simulink model "framework_sim_r2018b"  (R2018b)
settings: Solver=FixedStepAuto  SolverName=FixedStepDiscrete  StartTime=T0  StopTime=Tf  FixedStep=Ts  EnableMultiTasking=on
model workspace (MAT data in the model file):
  aKalman = Simulink.Parameter
  aKalman.DataType = 'auto'
  aKalman.Dimensions = [0 0]
  slipEnabler = Simulink.Parameter
  slipEnabler.DataType = 'auto'
  slipEnabler.Dimensions = [0 0]
values from neighbouring files (symbols this model uses):
  enable_onlinePlots = 0    [main_framework.m]
  enable_zoom = 1    [main_framework.m]
  LLC_sampleTime = LLC.sample_time    [main_framework.m]
  longCTRparam = longitController()    [main_framework.m]
  mapObjects = scenario.scenario_data.mapObjects    [main_framework.m]
  pacejkaParam = loadPacejkaParam()    [main_framework.m]
  refRoute_fewPoints = referencePath_fewPoints.refRoute_fewPoints    [main_framework.m]
  tau_D = vehicle_data.steering_system.tau_D    [main_framework.m]
  Ts = simulationPars.times.step_size    [main_framework.m]
  vehicle_data = getVehicleDataStruct()    [main_framework.m]
  X0 = loadInitialConditions    [main_framework.m]
undefined symbols (not defined in the file or in its folder): DiscIntNeverNeededParam, latContr_select
libraries: simulink_extras x13, drivingvehiclecontroller x2, simulink x1
settings Model: Creator=Edoardo  LastModifiedBy=tonegas
settings DataIOCC: SaveFormat=Array  ReturnWorkspaceOutputs=on
settings OptimizationCC: DefaultParameterBehavior=Inlined  PassReuseOutputArgsAs=Individual arguments  MaxStackSize=64
settings DebuggingCC: ReadBeforeWriteMsg=DisableAll  WriteAfterWriteMsg=DisableAll  WriteAfterReadMsg=DisableAll  MultiTaskDSMMsg=none  ParameterTunabilityLossMsg=error  SFUnexpectedBacktrackingDiag=warning  SFNoUnconditionalDefaultTransitionDiag=warning  SFExecutionAtInitializationDiag=none
settings HardwareCC: ProdBitPerInt=16  ProdBitPerPointer=16  ProdBitPerSizeT=16  ProdBitPerPtrDiffT=16  ProdLargestAtomicFloat=None  ProdWordSize=16  ProdHWDeviceType=STMicroelectronics->ST10/Super10
settings ModelReferenceCC: UpdateModelReferenceTargets=IfOutOfDate  PropagateSignalLabelsOutOfModel=off
settings SFSimCC: SFSimEcho=off  SimUseLocalCustomCode=off  MATLABDynamicMemAlloc=off
settings RTWCC: SystemTargetFile=ert.tlc  TemplateMakefile=ert_default_tmf  GenerateReport=on  RetainRTWFile=on  RTWUseLocalCustomCode=off  Toolchain=GNU Tools for ARM Embedded Processors  BuildConfiguration=Faster Runs  IncludeHyperlinkInReport=on  LaunchReport=on  GenerateTraceInfo=on  GenerateTraceReport=on  GenerateTraceReportSl=on  GenerateTraceReportSf=on  GenerateTraceReportEml=on
settings CodeAppCC: ForceParamTrailComments=on  IgnoreCustomStorageClasses=off  OperatorAnnotations=on  SimulinkDataObjDesc=on  SFDataObjDesc=on  InsertBlockDesc=on
settings ERTTargetCC: CodeReplacementLibrary=ARM Cortex-M (Optimized)  SupportVariableSizeSignals=on  RootIOFormat=Structure reference  ERTCustomFileTemplate=example_file_process.tlc
settings ConfigComp: CovMetricSettings=dw  CovSaveCumulativeToWorkspaceVar=on  CovSaveSingleToWorkspaceVar=on  CovExternalEMLEnable=off

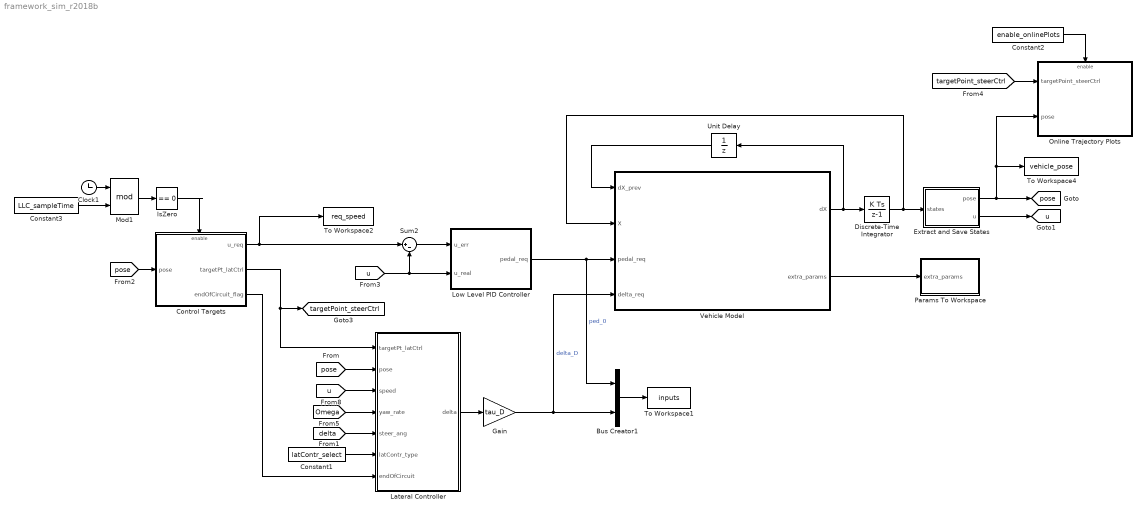
== system framework_sim_r2018b ==
  Bus Creator1 : BusCreator  Inputs=2
  Clock1 : Clock
  Constant1 : Constant  Value=latContr_select
  Constant2 : Constant  Value=enable_onlinePlots
  Constant3 : Constant  Value=LLC_sampleTime
  Control Targets : Subsystem
  Discrete-Time Integrator : DiscreteIntegrator  gainval=1  InitialCondition=X0  SampleTime=-1  ICPrevOutput=DiscIntNeverNeededParam  ICPrevScaledInput=DiscIntNeverNeededParam
  Extract and Save States : Subsystem
  Gain : Gain  Gain=tau_D
  IsZero : simulink/Logic and Bit Operations/Compare To Zero  relop===  OutDataTypeStr=boolean
  Lateral Controller : Subsystem
  Low Level PID Controller : Subsystem
  Mod1 : Math  Operator=mod  SaturateOnIntegerOverflow=on
  Online Trajectory Plots : Subsystem
      mask Display: image('example_path.png'); % Use "Edit Image" on toolstrip to change.
  Params To Workspace : Subsystem
  Sum2 : Sum  Inputs=|+-
  To Workspace1 : ToWorkspace  VariableName=inputs  SaveFormat=Timeseries  SampleTime=-1
  To Workspace2 : ToWorkspace  VariableName=req_speed  SaveFormat=Timeseries  SampleTime=-1
  To Workspace4 : ToWorkspace  VariableName=vehicle_pose  SampleTime=-1
      settings: Save2DSignal=2-D array (concatenate along first dimension)
  Unit Delay : UnitDelay  InitialCondition=zeros(size(X0))  SampleTime=-1  HasFrameUpgradeWarning=on
  Vehicle Model : MATLAB Function  TreatAsAtomicUnit=on
  tag scope: pose=global, targetPoint_steerCtrl=global, u=global
  wires:
  [targetPoint_steerCtrl] -> Online Trajectory Plots/1(targetPoint_steerCtrl)
  Constant2/1 -> Online Trajectory Plots/Enable
  [pose] -> Lateral Controller/2(pose)
  [u] -> Lateral Controller/3(speed)
  Constant1/1 -> Lateral Controller/6(latContr_type)
  [Omega] -> Lateral Controller/4(yaw_rate)
  [delta] -> Lateral Controller/5(steer_ang)
  Control Targets/2(targetPt_latCtrl) -> Lateral Controller/1(targetPt_latCtrl), [targetPoint_steerCtrl]
  [pose] -> Control Targets/1(pose)
  Clock1/1 -> Mod1/1
  Constant3/1 -> Mod1/2
  Mod1/1 -> IsZero/1
  IsZero/1 -> Control Targets/Enable
  Control Targets/3(endOfCircuit_flag) -> Lateral Controller/7(endOfCircuit)
  Unit Delay/1 -> Vehicle Model/1(dX_prev)
  Discrete-Time Integrator/1 -> Extract and Save States/1(states), Vehicle Model/2(X)
  Sum2/1 -> Low Level PID Controller/1(u_err)
  Gain/1 -> Bus Creator1/2, Vehicle Model/4(delta_req)  "delta_D"
  Control Targets/1(u_req) -> Sum2/1, To Workspace2/1
  Vehicle Model/1(dX) -> Unit Delay/1, Discrete-Time Integrator/1
  Vehicle Model/2(extra_params) -> Params To Workspace/1(extra_params)
  Bus Creator1/1 -> To Workspace1/1
  Low Level PID Controller/1(pedal_req) -> Vehicle Model/3(pedal_req), Bus Creator1/1  "ped_0"
  Lateral Controller/1(delta) -> Gain/1
  Extract and Save States/1(pose) -> [pose], Online Trajectory Plots/2(pose), To Workspace4/1
  Extract and Save States/2(u) -> [u]
  [u] -> Sum2/2, Low Level PID Controller/2(u_real)

== system framework_sim_r2018b/Control Targets ==
  pose : Inport
  Enable : EnablePort
  MATLAB System : MATLABSystem  System=setControlTargets  lateralController_type=latContr_select  purePursuit_lookAhead=purePursuitParams.lookAhead  clothoidBased_lookAhead=clothoidBasedParams.lookAhead  refRoute_points=refRoute_fewPoints  Lf=vehicle_data.vehicle.Lf  x_parkLot=mapObjects(1,1)  y_lowBound_parkLot=mapObjects(2,2)  y_uppBound_parkLot=mapObjects(1,2)  SimulateUsing=Interpreted execution
      mask Type: setControlTargets
      mask Display:
      | disp('setControlTargets');
      | port_label('input',1,'vehPose');
      | port_label('output',1,'targetPoint_latControl');
      | port_label('output',2,'speed_req');
      | port_label('output',3,'endOfCircuit');
  u_req : Outport  VectorParamsAs1DForOutWhenUnconnected=off
  targetPt_latCtrl : Outport  Port=2  VectorParamsAs1DForOutWhenUnconnected=off
  endOfCircuit_flag : Outport  Port=3  VectorParamsAs1DForOutWhenUnconnected=off
  wires:
  pose/1 -> MATLAB System/1
  MATLAB System/2 -> u_req/1
  MATLAB System/1 -> targetPt_latCtrl/1
  MATLAB System/3 -> endOfCircuit_flag/1

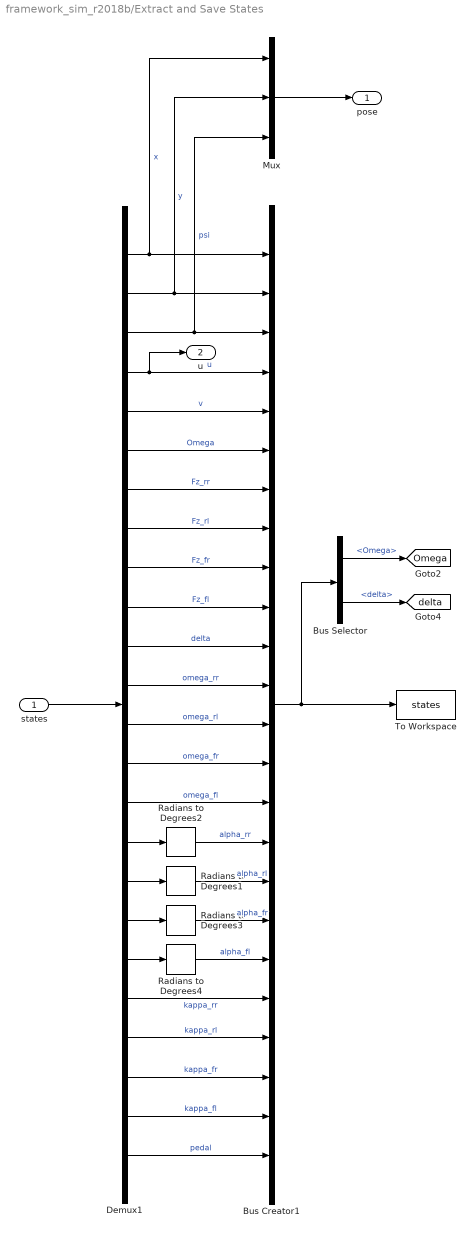
== system framework_sim_r2018b/Extract and Save States ==
  states : Inport
  Bus Creator1 : BusCreator  Inputs=24
  Bus Selector : BusSelector  OutputSignals=Omega,delta
  Demux1 : Demux  Outputs=24
  Mux : Mux  Inputs=3
  Radians to Degrees{1..4} (4 alike) : simulink_extras/Transformations/Radians to Degrees
  To Workspace : ToWorkspace  VariableName=states  SaveFormat=Timeseries  SampleTime=-1
  pose : Outport
  u : Outport  Port=2
  tag scope: Omega=global, delta=global
  wires:
  Demux1/13 -> Bus Creator1/13  "omega_rl"
  Demux1/8 -> Bus Creator1/8  "Fz_rl"
  Demux1/23 -> Bus Creator1/23  "kappa_fl"
  Demux1/19 -> Radians to Degrees4/1
  states/1 -> Demux1/1
  Demux1/14 -> Bus Creator1/14  "omega_fr"
  Demux1/7 -> Bus Creator1/7  "Fz_rr"
  Demux1/15 -> Bus Creator1/15  "omega_fl"
  Demux1/3 -> Mux/3, Bus Creator1/3  "psi"
  Demux1/22 -> Bus Creator1/22  "kappa_fr"
  Demux1/4 -> Bus Creator1/4, u/1  "u"
  Demux1/6 -> Bus Creator1/6  "Omega"
  Demux1/11 -> Bus Creator1/11  "delta"
  Demux1/5 -> Bus Creator1/5  "v"
  Demux1/9 -> Bus Creator1/9  "Fz_fr"
  Demux1/21 -> Bus Creator1/21  "kappa_rl"
  Demux1/12 -> Bus Creator1/12  "omega_rr"
  Demux1/17 -> Radians to Degrees1/1
  Demux1/2 -> Mux/2, Bus Creator1/2  "y"
  Demux1/20 -> Bus Creator1/20  "kappa_rr"
  Demux1/10 -> Bus Creator1/10  "Fz_fl"
  Demux1/18 -> Radians to Degrees3/1
  Demux1/1 -> Mux/1, Bus Creator1/1  "x"
  Demux1/16 -> Radians to Degrees2/1
  Bus Creator1/1 -> Bus Selector/1, To Workspace/1
  Radians to Degrees2/1 -> Bus Creator1/16  "alpha_rr"
  Radians to Degrees1/1 -> Bus Creator1/17  "alpha_rl"
  Radians to Degrees3/1 -> Bus Creator1/18  "alpha_fr"
  Radians to Degrees4/1 -> Bus Creator1/19  "alpha_fl"
  Demux1/24 -> Bus Creator1/24  "pedal"
  Mux/1 -> pose/1
  Bus Selector/1 -> [Omega]  "<Omega>"
  Bus Selector/2 -> [delta]  "<delta>"

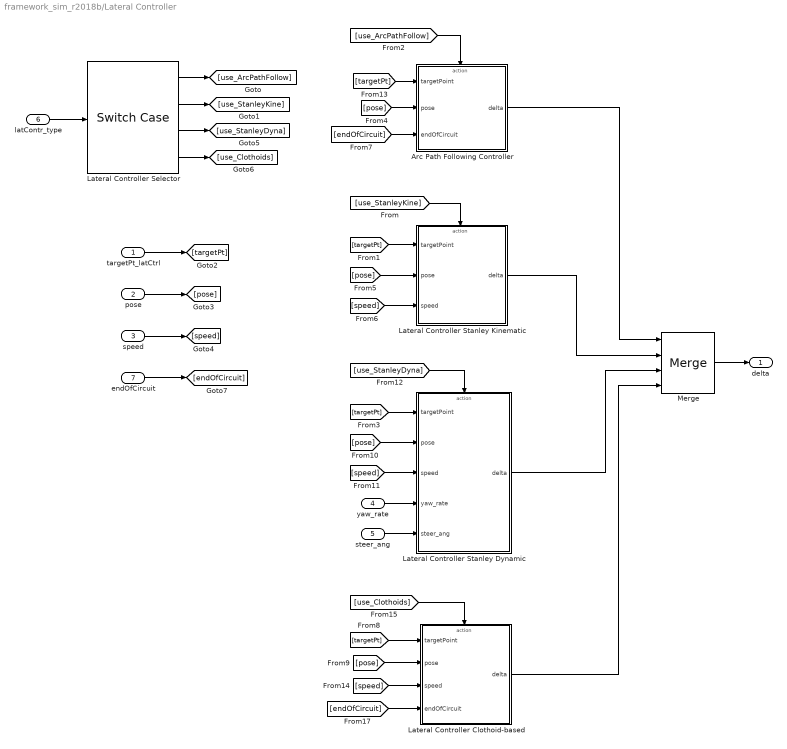
== system framework_sim_r2018b/Lateral Controller ==
  targetPt_latCtrl : Inport
  pose : Inport  Port=2
  speed : Inport  Port=3
  yaw_rate : Inport  Port=4
  steer_ang : Inport  Port=5
  latContr_type : Inport  Port=6
  endOfCircuit : Inport  Port=7
  Arc Path Following Controller : Subsystem  TreatAsAtomicUnit=on
  Lateral Controller Clothoid-based : Subsystem  TreatAsAtomicUnit=on
  Lateral Controller Selector : SwitchCase  CaseConditions={1,2,3,4}  ShowDefaultCase=off
  Lateral Controller Stanley Dynamic : Subsystem  TreatAsAtomicUnit=on
  Lateral Controller Stanley Kinematic : Subsystem  TreatAsAtomicUnit=on
  Merge : Merge  Inputs=4
  delta : Outport  VectorParamsAs1DForOutWhenUnconnected=off
  wires:
  Arc Path Following Controller/1(delta) -> Merge/1
  latContr_type/1 -> Lateral Controller Selector/1
  Lateral Controller Stanley Kinematic/1(delta) -> Merge/2
  Merge/1 -> delta/1
  Lateral Controller Selector/1 -> [use_ArcPathFollow]
  [use_ArcPathFollow] -> Arc Path Following Controller/Action
  Lateral Controller Selector/2 -> [use_StanleyKine]
  [use_StanleyKine] -> Lateral Controller Stanley Kinematic/Action
  targetPt_latCtrl/1 -> [targetPt]
  [targetPt] -> Arc Path Following Controller/1(targetPoint)
  [targetPt] -> Lateral Controller Stanley Kinematic/1(targetPoint)
  pose/1 -> [pose]
  [pose] -> Arc Path Following Controller/2(pose)
  [pose] -> Lateral Controller Stanley Kinematic/2(pose)
  speed/1 -> [speed]
  [speed] -> Lateral Controller Stanley Kinematic/3(speed)
  Lateral Controller Selector/3 -> [use_StanleyDyna]
  [pose] -> Lateral Controller Stanley Dynamic/2(pose)
  [targetPt] -> Lateral Controller Stanley Dynamic/1(targetPoint)
  [speed] -> Lateral Controller Stanley Dynamic/3(speed)
  [use_StanleyDyna] -> Lateral Controller Stanley Dynamic/Action
  Lateral Controller Stanley Dynamic/1(delta) -> Merge/3
  yaw_rate/1 -> Lateral Controller Stanley Dynamic/4(yaw_rate)
  steer_ang/1 -> Lateral Controller Stanley Dynamic/5(steer_ang)
  [use_Clothoids] -> Lateral Controller Clothoid-based/Action
  [pose] -> Lateral Controller Clothoid-based/2(pose)
  [targetPt] -> Lateral Controller Clothoid-based/1(targetPoint)
  [speed] -> Lateral Controller Clothoid-based/3(speed)
  Lateral Controller Clothoid-based/1(delta) -> Merge/4
  Lateral Controller Selector/4 -> [use_Clothoids]
  [endOfCircuit] -> Arc Path Following Controller/3(endOfCircuit)
  [endOfCircuit] -> Lateral Controller Clothoid-based/4(endOfCircuit)
  endOfCircuit/1 -> [endOfCircuit]

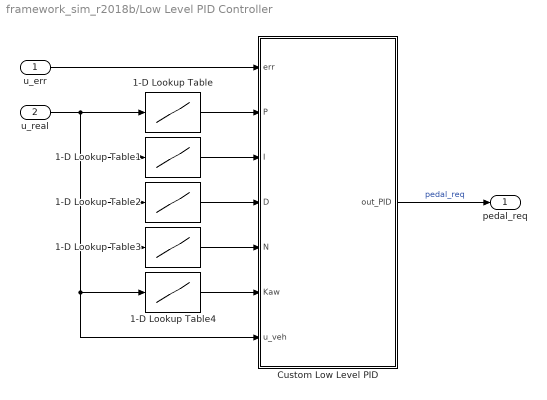
== system framework_sim_r2018b/Low Level PID Controller ==
  u_err : Inport
  u_real : Inport  Port=2
  1-D Lookup Table : Lookup_n-D  NumberOfTableDimensions=1  BreakpointsForDimension1=longCTRparam.speed_vals_PID_sched  BeginIndexSearchUsingPreviousIndexResult=on  Table=longCTRparam.Kp_vals  ExtrapMethod=Clip  UseLastTableValue=on  InternalRulePriority=Speed  RndMeth=Simplest  InputSameDT=on
  1-D Lookup Table1 : Lookup_n-D  NumberOfTableDimensions=1  BreakpointsForDimension1=longCTRparam.speed_vals_PID_sched  BeginIndexSearchUsingPreviousIndexResult=on  Table=longCTRparam.Ki_vals  ExtrapMethod=Clip  UseLastTableValue=on  InternalRulePriority=Speed  RndMeth=Simplest  InputSameDT=on
  1-D Lookup Table2 : Lookup_n-D  NumberOfTableDimensions=1  BreakpointsForDimension1=longCTRparam.speed_vals_PID_sched  BeginIndexSearchUsingPreviousIndexResult=on  Table=longCTRparam.Kd_vals  ExtrapMethod=Clip  UseLastTableValue=on  InternalRulePriority=Speed  RndMeth=Simplest  InputSameDT=on
  1-D Lookup Table3 : Lookup_n-D  NumberOfTableDimensions=1  BreakpointsForDimension1=longCTRparam.speed_vals_PID_sched  BeginIndexSearchUsingPreviousIndexResult=on  Table=longCTRparam.N_vals  ExtrapMethod=Clip  UseLastTableValue=on  InternalRulePriority=Speed  RndMeth=Simplest  InputSameDT=on
  1-D Lookup Table4 : Lookup_n-D  NumberOfTableDimensions=1  BreakpointsForDimension1=longCTRparam.speed_vals_PID_sched  BeginIndexSearchUsingPreviousIndexResult=on  Table=longCTRparam.Kaw_vals  ExtrapMethod=Clip  UseLastTableValue=on  InternalRulePriority=Speed  RndMeth=Simplest  InputSameDT=on
  Custom Low Level PID : Subsystem
  pedal_req : Outport  VectorParamsAs1DForOutWhenUnconnected=off
  wires:
  1-D Lookup Table/1 -> Custom Low Level PID/2(P)
  u_err/1 -> Custom Low Level PID/1(err)
  u_real/1 -> 1-D Lookup Table4/1, Custom Low Level PID/7(u_veh), 1-D Lookup Table3/1, 1-D Lookup Table2/1, 1-D Lookup Table1/1, 1-D Lookup Table/1
  1-D Lookup Table2/1 -> Custom Low Level PID/4(D)
  1-D Lookup Table3/1 -> Custom Low Level PID/5(N)
  1-D Lookup Table1/1 -> Custom Low Level PID/3(I)
  Custom Low Level PID/1(out_PID) -> pedal_req/1  "pedal_req"
  1-D Lookup Table4/1 -> Custom Low Level PID/6(Kaw)

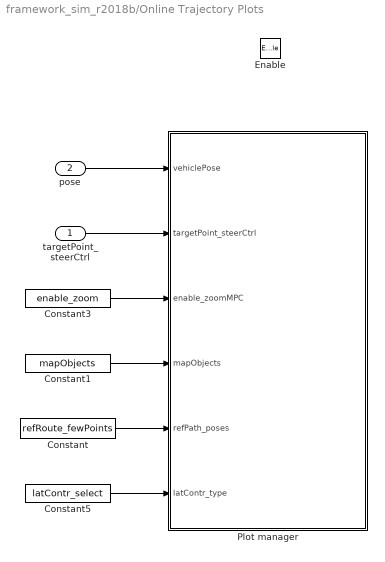
== system framework_sim_r2018b/Online Trajectory Plots ==
  targetPoint_steerCtrl : Inport
  pose : Inport  Port=2
  Enable : EnablePort
  Constant : Constant  Value=refRoute_fewPoints
  Constant1 : Constant  Value=mapObjects
  Constant3 : Constant  Value=enable_zoom
  Constant5 : Constant  Value=latContr_select
  Plot manager : MATLAB Function  TreatAsAtomicUnit=on
  wires:
  Constant1/1 -> Plot manager/4(mapObjects)
  targetPoint_steerCtrl/1 -> Plot manager/2(targetPoint_steerCtrl)
  Constant5/1 -> Plot manager/6(latContr_type)
  Constant/1 -> Plot manager/5(refPath_poses)
  pose/1 -> Plot manager/1(vehiclePose)
  Constant3/1 -> Plot manager/3(enable_zoomMPC)

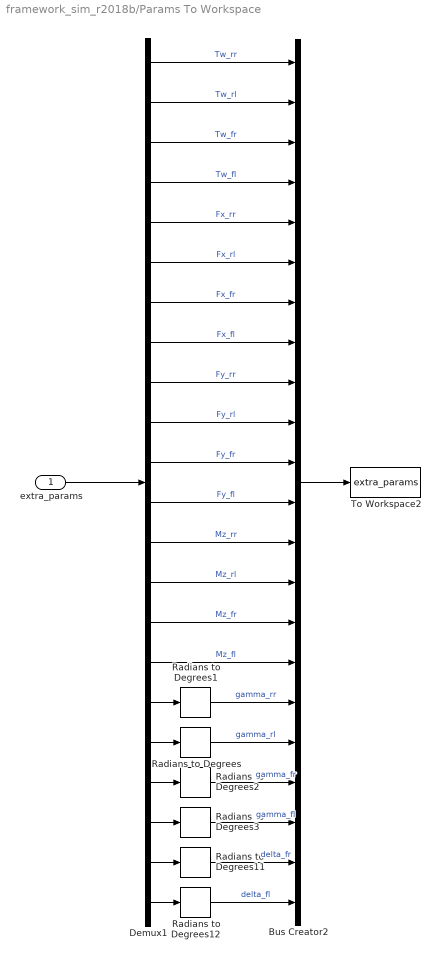
== system framework_sim_r2018b/Params To Workspace ==
  extra_params : Inport
  Bus Creator2 : BusCreator  Inputs=22
  Demux1 : Demux  Outputs=22
  Radians to Degrees{,1..3,11..12} (6 alike) : simulink_extras/Transformations/Radians to Degrees
  To Workspace2 : ToWorkspace  VariableName=extra_params  SaveFormat=Timeseries  SampleTime=-1
  wires:
  Demux1/17 -> Radians to Degrees1/1
  Demux1/3 -> Bus Creator2/3  "Tw_fr"
  Radians to Degrees3/1 -> Bus Creator2/20  "gamma_fl"
  Demux1/16 -> Bus Creator2/16  "Mz_fl"
  Radians to Degrees1/1 -> Bus Creator2/17  "gamma_rr"
  Radians to Degrees11/1 -> Bus Creator2/21  "delta_fr"
  Demux1/14 -> Bus Creator2/14  "Mz_rl"
  Demux1/4 -> Bus Creator2/4  "Tw_fl"
  Demux1/6 -> Bus Creator2/6  "Fx_rl"
  Demux1/8 -> Bus Creator2/8  "Fx_fl"
  Demux1/13 -> Bus Creator2/13  "Mz_rr"
  Demux1/7 -> Bus Creator2/7  "Fx_fr"
  Demux1/5 -> Bus Creator2/5  "Fx_rr"
  Demux1/9 -> Bus Creator2/9  "Fy_rr"
  Demux1/11 -> Bus Creator2/11  "Fy_fr"
  Demux1/15 -> Bus Creator2/15  "Mz_fr"
  Demux1/10 -> Bus Creator2/10  "Fy_rl"
  Radians to Degrees12/1 -> Bus Creator2/22  "delta_fl"
  Radians to Degrees2/1 -> Bus Creator2/19  "gamma_fr"
  extra_params/1 -> Demux1/1
  Demux1/12 -> Bus Creator2/12  "Fy_fl"
  Bus Creator2/1 -> To Workspace2/1
  Demux1/1 -> Bus Creator2/1  "Tw_rr"
  Demux1/2 -> Bus Creator2/2  "Tw_rl"
  Radians to Degrees/1 -> Bus Creator2/18  "gamma_rl"
  Demux1/18 -> Radians to Degrees/1
  Demux1/19 -> Radians to Degrees2/1
  Demux1/20 -> Radians to Degrees3/1
  Demux1/21 -> Radians to Degrees11/1
  Demux1/22 -> Radians to Degrees12/1

== system framework_sim_r2018b/Lateral Controller/Arc Path Following Controller ==
  targetPoint : Inport
  pose : Inport  Port=2
  endOfCircuit : Inport  Port=3
  Action Port : ActionPort
  Arc Path Following Controller : MATLAB Function  TreatAsAtomicUnit=on
  delta : Outport  VectorParamsAs1DForOutWhenUnconnected=off
  wires:
  Arc Path Following Controller/1(delta) -> delta/1
  targetPoint/1 -> Arc Path Following Controller/1(target_Point)
  pose/1 -> Arc Path Following Controller/2(pose)
  endOfCircuit/1 -> Arc Path Following Controller/3(endOfCircuit)

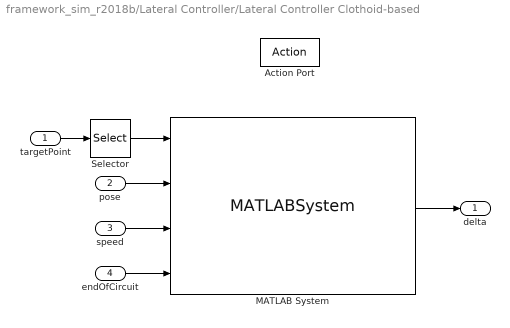
== system framework_sim_r2018b/Lateral Controller/Lateral Controller Clothoid-based ==
  targetPoint : Inport
  pose : Inport  Port=2
  speed : Inport  Port=3
  endOfCircuit : Inport  Port=4
  Action Port : ActionPort
  MATLAB System : MATLABSystem  System=clothoidBased_lateralController  lookAhead=clothoidBasedParams.lookAhead  Kus=clothoidBasedParams.Kus  L=vehicle_data.vehicle.L  SimulateUsing=Interpreted execution
      mask Type: clothoidBased_lateralController
      mask Display:
      | disp('clothoidBased_lateralController');
      | port_label('input',1,'targetPoint');
      | port_label('input',2,'vehPose');
      | port_label('input',3,'vehSpeed');
      | port_label('input',4,'endOfCircuit');
      | port_label('output',1,'delta_req');
  Selector : Selector  InputPortWidth=4  IndexOptions=Index vector (dialog)  Indices=[1 2 3]  OutputSizes=1
  delta : Outport  VectorParamsAs1DForOutWhenUnconnected=off
  wires:
  speed/1 -> MATLAB System/3
  MATLAB System/1 -> delta/1
  pose/1 -> MATLAB System/2
  targetPoint/1 -> Selector/1
  Selector/1 -> MATLAB System/1
  endOfCircuit/1 -> MATLAB System/4

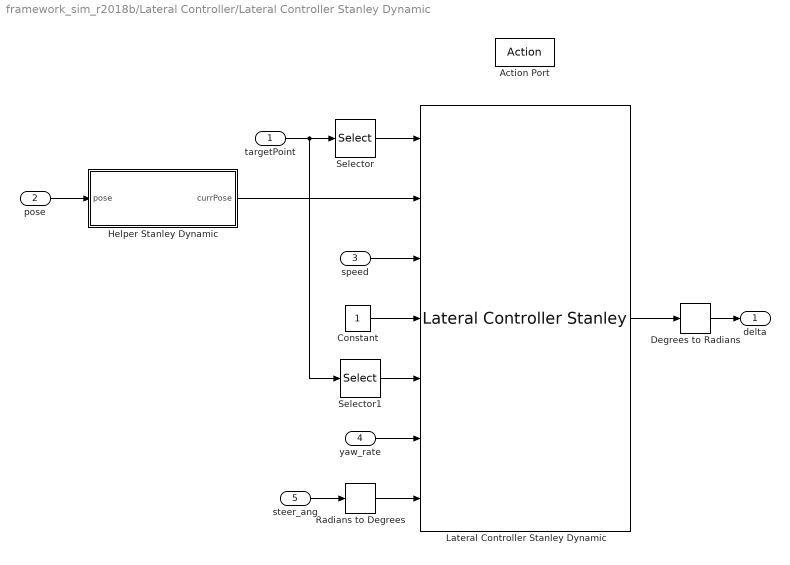
== system framework_sim_r2018b/Lateral Controller/Lateral Controller Stanley Dynamic ==
  targetPoint : Inport
  pose : Inport  Port=2
  speed : Inport  Port=3
  yaw_rate : Inport  Port=4
  steer_ang : Inport  Port=5
  Action Port : ActionPort
  Constant : Constant
  Degrees to Radians : simulink_extras/Transformations/Degrees to Radians
  Helper Stanley Dynamic : MATLAB Function  TreatAsAtomicUnit=on
  Lateral Controller Stanley Dynamic : drivingvehiclecontroller/Lateral Controller Stanley  ModelType=Dynamic bicycle model  PositionGainF=stanleyParams.positGainFW  PositionGainR=stanleyParams.positGainREV  YawRateGain=stanleyParams.yawRateGain  DelayGain=stanleyParams.steerGain  VehicleMass=vehicle_data.vehicle.m  Lf=vehicle_data.vehicle.Lf  Lr=vehicle_data.vehicle.Lr  TireStiffness=stanleyParams.cornerStiff  Wheelbase=2.8  MaxSteeringAngle=stanleyParams.maxSteerAngle
      settings: SourceProductBaseCode=DR
  Radians to Degrees : simulink_extras/Transformations/Radians to Degrees
  Selector : Selector  InputPortWidth=4  IndexOptions=Index vector (dialog)  Indices=[1 2 3]  OutputSizes=1
  Selector1 : Selector  InputPortWidth=4  IndexOptions=Index vector (dialog)  Indices=[4]  OutputSizes=1
  delta : Outport  VectorParamsAs1DForOutWhenUnconnected=off
  wires:
  Lateral Controller Stanley Dynamic/1 -> Degrees to Radians/1
  pose/1 -> Helper Stanley Dynamic/1(pose)
  speed/1 -> Lateral Controller Stanley Dynamic/3
  Constant/1 -> Lateral Controller Stanley Dynamic/4
  Degrees to Radians/1 -> delta/1
  Helper Stanley Dynamic/1(currPose) -> Lateral Controller Stanley Dynamic/2
  targetPoint/1 -> Selector1/1, Selector/1
  Selector/1 -> Lateral Controller Stanley Dynamic/1
  Selector1/1 -> Lateral Controller Stanley Dynamic/5
  yaw_rate/1 -> Lateral Controller Stanley Dynamic/6
  Radians to Degrees/1 -> Lateral Controller Stanley Dynamic/7
  steer_ang/1 -> Radians to Degrees/1

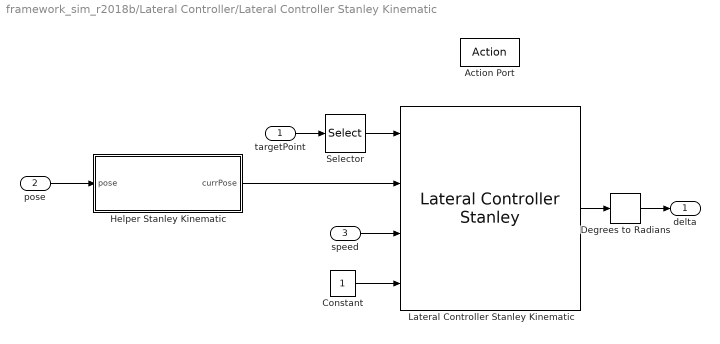
== system framework_sim_r2018b/Lateral Controller/Lateral Controller Stanley Kinematic ==
  targetPoint : Inport
  pose : Inport  Port=2
  speed : Inport  Port=3
  Action Port : ActionPort
  Constant : Constant
  Degrees to Radians : simulink_extras/Transformations/Degrees to Radians
  Helper Stanley Kinematic : MATLAB Function  TreatAsAtomicUnit=on
  Lateral Controller Stanley Kinematic : drivingvehiclecontroller/Lateral Controller Stanley  ModelType=Kinematic bicycle model  PositionGainF=stanleyParams.positGainFW  PositionGainR=stanleyParams.positGainREV  YawRateGain=0.2  DelayGain=0.2  VehicleMass=1575  Lf=1.2  Lr=1.6  TireStiffness=19000  Wheelbase=vehicle_data.vehicle.Lf + vehicle_data.vehicle.Lr  MaxSteeringAngle=stanleyParams.maxSteerAngle
      settings: SourceProductBaseCode=DR
  Selector : Selector  InputPortWidth=4  IndexOptions=Index vector (dialog)  Indices=[1 2 3]  OutputSizes=1
  delta : Outport  VectorParamsAs1DForOutWhenUnconnected=off
  wires:
  Lateral Controller Stanley Kinematic/1 -> Degrees to Radians/1
  pose/1 -> Helper Stanley Kinematic/1(pose)
  speed/1 -> Lateral Controller Stanley Kinematic/3
  Constant/1 -> Lateral Controller Stanley Kinematic/4
  Degrees to Radians/1 -> delta/1
  Helper Stanley Kinematic/1(currPose) -> Lateral Controller Stanley Kinematic/2
  targetPoint/1 -> Selector/1
  Selector/1 -> Lateral Controller Stanley Kinematic/1

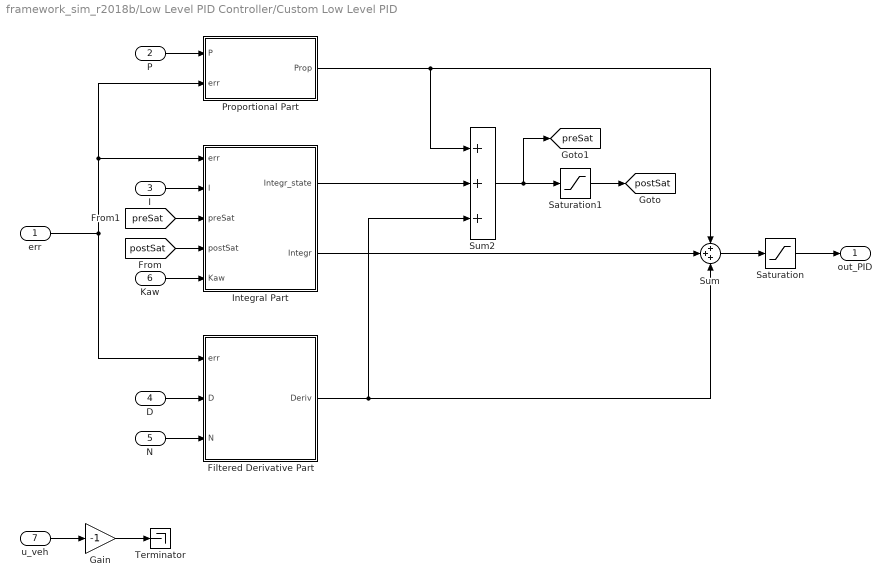
== system framework_sim_r2018b/Low Level PID Controller/Custom Low Level PID ==
  err : Inport
  P : Inport  Port=2
  I : Inport  Port=3
  D : Inport  Port=4
  N : Inport  Port=5
  Kaw : Inport  Port=6
  u_veh : Inport  Port=7
  Filtered Derivative Part : Subsystem
  Gain : Gain  Gain=-1
  Integral Part : Subsystem
  Proportional Part : Subsystem
  Saturation : Saturate  UpperLimit=1  LowerLimit=-1  LinearizeAsGain=off
  Saturation1 : Saturate  UpperLimit=1  LowerLimit=-1  LinearizeAsGain=off
  Sum : Sum  Inputs=+++
  Sum2 : Sum  Inputs=+++
  Terminator : Terminator
  out_PID : Outport  VectorParamsAs1DForOutWhenUnconnected=off
  tag scope: postSat=global, preSat=global
  wires:
  Sum2/1 -> [preSat], Saturation1/1
  Sum/1 -> Saturation/1
  Saturation/1 -> out_PID/1
  err/1 -> Filtered Derivative Part/1(err), Proportional Part/2(err), Integral Part/1(err)
  Saturation1/1 -> [postSat]
  I/1 -> Integral Part/2(I)
  Integral Part/1(Integr_state) -> Sum2/2
  Integral Part/2(Integr) -> Sum/2
  Proportional Part/1(Prop) -> Sum2/1, Sum/1
  P/1 -> Proportional Part/1(P)
  [preSat] -> Integral Part/3(preSat)
  [postSat] -> Integral Part/4(postSat)
  Filtered Derivative Part/1(Deriv) -> Sum/3, Sum2/3
  D/1 -> Filtered Derivative Part/2(D)
  N/1 -> Filtered Derivative Part/3(N)
  u_veh/1 -> Gain/1
  Gain/1 -> Terminator/1
  Kaw/1 -> Integral Part/5(Kaw)

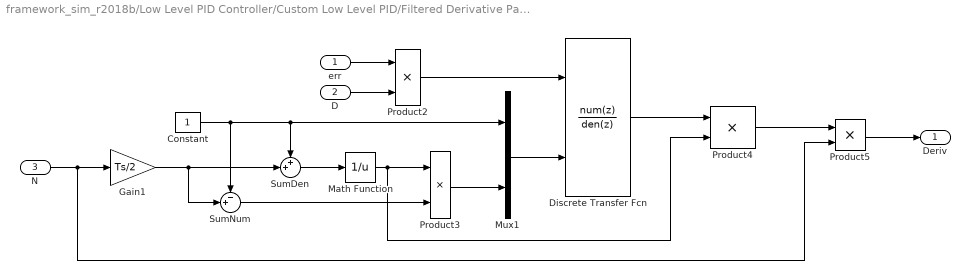
== system framework_sim_r2018b/Low Level PID Controller/Custom Low Level PID/Filtered Derivative Part ==
  err : Inport
  D : Inport  Port=2
  N : Inport  Port=3
  Constant : Constant
  Discrete Transfer Fcn : DiscreteTransferFcn  Numerator=[1 -1]  DenominatorSource=Input port  SampleTime=Ts  a0EqualsOne=on
      settings: InputPortMap=u0,p3
  Gain1 : Gain  Gain=Ts/2
  Math Function : Math  Operator=reciprocal  SaturateOnIntegerOverflow=on
  Mux1 : Mux  Inputs=2
  Product{2..5} (4 alike) : Product
  SumDen : Sum  Inputs=++|
  SumNum : Sum  Inputs=-+|
  Deriv : Outport  VectorParamsAs1DForOutWhenUnconnected=off
  wires:
  N/1 -> Gain1/1, Product5/2
  Product4/1 -> Product5/1
  SumDen/1 -> Math Function/1
  Math Function/1 -> Product4/2, Product3/1
  SumNum/1 -> Product3/2
  Product2/1 -> Discrete Transfer Fcn/1
  Discrete Transfer Fcn/1 -> Product4/1
  Constant/1 -> SumNum/1, SumDen/1, Mux1/1
  Product3/1 -> Mux1/2
  Mux1/1 -> Discrete Transfer Fcn/2
  Gain1/1 -> SumNum/2, SumDen/2
  err/1 -> Product2/1
  D/1 -> Product2/2
  Product5/1 -> Deriv/1

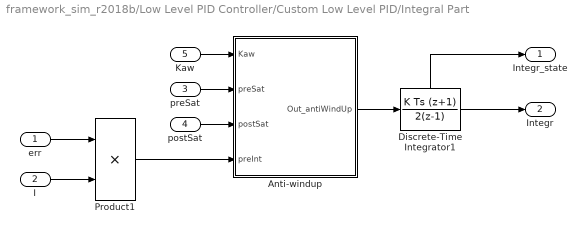
== system framework_sim_r2018b/Low Level PID Controller/Custom Low Level PID/Integral Part ==
  err : Inport
  I : Inport  Port=2
  preSat : Inport  Port=3
  postSat : Inport  Port=4
  Kaw : Inport  Port=5
  Anti-windup : Subsystem
  Discrete-Time Integrator1 : DiscreteIntegrator  IntegratorMethod=Integration: Trapezoidal  SampleTime=Ts  ShowStatePort=on  ICPrevOutput=DiscIntNeverNeededParam  ICPrevScaledInput=DiscIntNeverNeededParam
  Product1 : Product
  Integr_state : Outport  VectorParamsAs1DForOutWhenUnconnected=off
  Integr : Outport  Port=2  VectorParamsAs1DForOutWhenUnconnected=off
  wires:
  Discrete-Time Integrator1/State -> Integr_state/1
  preSat/1 -> Anti-windup/2(preSat)
  Product1/1 -> Anti-windup/4(preInt)
  postSat/1 -> Anti-windup/3(postSat)
  I/1 -> Product1/2
  Anti-windup/1(Out_antiWindUp) -> Discrete-Time Integrator1/1
  Discrete-Time Integrator1/1 -> Integr/1
  err/1 -> Product1/1
  Kaw/1 -> Anti-windup/1(Kaw)

== system framework_sim_r2018b/Low Level PID Controller/Custom Low Level PID/Proportional Part ==
  P : Inport
  err : Inport  Port=2
  Product : Product
  Prop : Outport  VectorParamsAs1DForOutWhenUnconnected=off
  wires:
  P/1 -> Product/2
  Product/1 -> Prop/1
  err/1 -> Product/1

== system framework_sim_r2018b/Low Level PID Controller/Custom Low Level PID/Integral Part/Anti-windup ==
  Kaw : Inport
  preSat : Inport  Port=2
  postSat : Inport  Port=3
  preInt : Inport  Port=4
  Product : Product
  Sum : Sum  Inputs=|-+
  Sum1 : Sum  Inputs=|++
  Out_antiWindUp : Outport  VectorParamsAs1DForOutWhenUnconnected=off
  wires:
  preSat/1 -> Sum/1
  preInt/1 -> Sum1/2
  Product/1 -> Sum1/1
  Sum1/1 -> Out_antiWindUp/1
  Sum/1 -> Product/2
  postSat/1 -> Sum/2
  Kaw/1 -> Product/1

== matlab function framework_sim_r2018b/Lateral Controller/Lateral Controller Stanley Dynamic/Helper Stanley Dynamic ==
  data: pose input; currPose output
function currPose = helperStanleyDyn(pose)

    currPose = [pose(1), pose(2), rad2deg(pose(3))];

end

== matlab function framework_sim_r2018b/Lateral Controller/Lateral Controller Stanley Kinematic/Helper Stanley Kinematic ==
  data: pose input; currPose output
function currPose = helperStanleyKine(pose)

    currPose = [pose(1), pose(2), rad2deg(pose(3))];

end

== matlab function framework_sim_r2018b/Online Trajectory Plots/Plot manager ==
  data: vehiclePose input; targetPoint_steerCtrl input; enable_zoomMPC input; mapObjects input; refPath_poses input; latContr_type input
function real_time_plot(vehiclePose,targetPoint_steerCtrl,enable_zoomMPC,mapObjects,refPath_poses,latContr_type)
    
    coder.extrinsic('patch');
    
    %% Extract vehicle pose
    xCoMCar = vehiclePose(1);
    yCoMCar = vehiclePose(2);
    vehicleAttitude = vehiclePose(3);
    
    %% Load vehicle data
    vehicle_data = getVehicleDataStruct();
    Lf = vehicle_data.vehicle.Lf;        
    Lr = vehicle_data.vehicle.Lr;                 
    Wf = vehicle_data.vehicle.Wf;     
    Wr = vehicle_data.vehicle.Wr;
    
    %% Delete the plots for the previous iteration
    cla;
    
    %% Sketch the vehicle and its position, for this MPC iteration
    % Rotation matrix from vehicle (mobile) frame to the absolute frame
    RotMat = [cos(vehicleAttitude), -sin(vehicleAttitude); ...
              sin(vehicleAttitude), cos(vehicleAttitude)];
    
    pos_vehRR = RotMat*[-Lr -Wr/2]';
    pos_vehRL = RotMat*[-Lr +Wr/2]';
    pos_vehFR = RotMat*[+Lf -Wf/2]';
    pos_vehFL = RotMat*[+Lf +Wf/2]';
    pos_veh   = [pos_vehRR pos_vehRL pos_vehFL pos_vehFR];
    
    % Current vehicle pose
    patch(xCoMCar + pos_veh(1,:),yCoMCar + pos_veh(2,:),'yellow');
    
    % Optimal route computed with route planner
    X_route = refPath_poses(:,1);
    Y_route = refPath_poses(:,2);
    plot(X_route,Y_route,'go','MarkerSize',2)
    
    % Objects of the road scenario (walls, fixed obstacles etc)
    for ii=1:size(mapObjects,1)
        rectangle('Position',mapObjects(ii,:),'FaceColor',color('purple'),'EdgeColor',color('purple'),'LineWidth',2)
    end
    
    % Target point used by some low-level lateral controllers
    if (latContr_type==1 || latContr_type==4)  
        plot(targetPoint_steerCtrl(1),targetPoint_steerCtrl(2),'r*','MarkerSize',6)
    end
    
    % Zoom on the vehicle if required
    if (enable_zoomMPC)
        xlim([xCoMCar-40 xCoMCar+40])
        ylim([yCoMCar-40 yCoMCar+40])
    end
    
end

== matlab function framework_sim_r2018b/Vehicle Model ==
  settings: sampleTime=step_size
  data: dX_prev input; X input; dX output; extra_params output; pedal_req input; delta_req input; pacejkaParam parameter; vehicle_data parameter
function [dX,extra_params] = Vehicle_model(dX_prev,X,pedal_req,delta_req,pacejkaParam,vehicle_data)

% ----------------------------------------------------------------
%% Double Track Vehicle Model of Formula SAE electric vehicle (Chimera Evoluzione)
%  authors: Mattia Piccinini & Gastone Pietro Papini Rosati
%  email:  mattia.piccinini@unitn.it
%  date:   13/10/2020
% ----------------------------------------------------------------


% ----------------------------------------------------------------
%% INPUTS OF THE MODEL
% ----------------------------------------------------------------

% Model inputs are: 
%       - requested pedal (throttle if >0, brake if <0)
%       - requested steering angle at the steering wheel delta_req (in [rad])


% ----------------------------------------------------------------
%% OUTPUTS OF THE MODEL
% ----------------------------------------------------------------

% The outputs of the model are the derivatives of all vehicle states,
% collected in the dX vector, as well as some other useful extra parameters 
% to describe vehicle behavior, saved in the extra_params vector

% Empty output vectors are here initialized 
dX = zeros(24,1);  
extra_params = zeros(22,1);  


% ----------------------------------------------------------------
%% STATES OF THE MODEL
% ----------------------------------------------------------------

x         = X(1);       % [m] x-coord of the vehicle CoM
y         = X(2);       % [m] y-coord of the vehicle CoM
psi       = X(3);       % [rad] yaw angle
u         = X(4);       % [m/s] vehicle longitudinal speed
v         = X(5);       % [m/s] vehicle lateral speed
Omega     = X(6);       % [rad/s] yaw rate
Fz__rr    = X(7);       % [N] vertical force for the rear right wheel
Fz__rl    = X(8);       % [N] vertical force for the rear left wheel
Fz__fr    = X(9);       % [N] vertical force for the front right wheel
Fz__fl    = X(10);      % [N] vertical force for the front left wheel
delta     = X(11);      % [rad] steering angle (at the wheel)
omega__rr = X(12);      % [rad/s] rotational speed rear right wheel
omega__rl = X(13);      % [rad/s] rotational speed rear left wheel 
omega__fr = X(14);      % [rad/s] rotational speed front right wheel 
omega__fl = X(15);      % [rad/s] rotational speed front left wheel 
alpha__rr = X(16);      % [rad] side slip angle rear right wheel
alpha__rl = X(17);      % [rad] side slip angle rear left wheel
alpha__fr = X(18);      % [rad] side slip angle front right wheel
alpha__fl = X(19);      % [rad] side slip angle front left wheel
kappa__rr = X(20);      % [-] longitudinal slip rear right wheel
kappa__rl = X(21);      % [-] longitudinal slip rear left wheel
kappa__fr = X(22);      % [-] longitudinal slip front right wheel
kappa__fl = X(23);      % [-] longitudinal slip front left wheel
ped       = X(24);      % [-] pedal

% ----------------------------------------------------------------
%% AUXILIARY MODELS
% ----------------------------------------------------------------

% ----------------------
% MOTOR MODEL
% ----------------------
% Driving torques at the wheels
Tm_req = posPart(ped)*vehicle_data.motor.maxTorque;
Tw__rr_traction = MotorModel(Tm_req,omega__rr,vehicle_data);
Tw__rl_traction = MotorModel(Tm_req,omega__rl,vehicle_data);
 
% ----------------------
% BRAKE MODEL
% ----------------------
Tb_r_req = -negPart(ped)*vehicle_data.braking.totBrakeTorque*(1-vehicle_data.braking.brakeRatio);
Tb_f_req = -negPart(ped)*vehicle_data.braking.totBrakeTorque*vehicle_data.braking.brakeRatio;
% Rear wheels braking model
[Tw__rr_brake,Tw__rl_brake] = brakeModelRear(Tb_r_req,omega__rr,omega__rl,vehicle_data); 
% Front wheels braking model
[Tw__fr_brake,Tw__fl_brake] = brakeModelFront(Tb_f_req,omega__fr,omega__fl,vehicle_data);

% ----------------------
% WHEEL TORQUES
% ----------------------
% The total torque for each wheel is the algebraic sum of motor and brake torques
Tw__rr = Tw__rr_traction + Tw__rr_brake;
Tw__rl = Tw__rl_traction + Tw__rl_brake;
Tw__fr = Tw__fr_brake;
Tw__fl = Tw__fl_brake;

% ----------------------
% CAMBER MODEL
% ----------------------
[gamma__rr, gamma__rl, gamma__fr, gamma__fl] = camberModel(vehicle_data);

% ----------------------
% ACKERMANN STEERING MODEL
% ----------------------
% Compute steering angles for front wheels, with perfect Ackerman steering model
[delta__fr, delta__fl] = perfectAcker(delta,vehicle_data);

% ----------------------
% LONGITUDINAL SLIPS
% ----------------------
% Longitudinal slip model including a correction for low speed 
[kappa__rr_corr,kappa__rl_corr,kappa__fr_corr,kappa__fl_corr] = longitSlipModel(u,Omega,kappa__rr,kappa__rl,kappa__fr,kappa__fl,omega__rr,omega__rl,omega__fr,omega__fl,delta__fr,delta__fl,Fz__rr,Fz__rl,Fz__fr,Fz__fl,gamma__rr,gamma__rl,gamma__fr,gamma__fl,pacejkaParam,vehicle_data);

% ----------------------
% AERODYNAMIC MODEL
% ----------------------
% Aero drag, downforce at rear axle, downforce at front axle
[FAxc, FAz__r, FAz__f] = aeroModel(u,vehicle_data);
          
% ----------------------
% TIRE PACEJKA MODEL
% ----------------------
% Ensure symmetric behavior of left and right tires by calculating the
% forces and moments for left tires via a previous change of sign of the
% side slip alpha and the camber gamma
[Fx__rr,Fy__rr,AM__rr] = pacejka_model(kappa__rr,Fz__rr,alpha__rr,gamma__rr,pacejkaParam);
[Fx__rl,Fy__rl,AM__rl] = pacejka_model(kappa__rl,Fz__rl,-alpha__rl,-gamma__rl,pacejkaParam);
[Fx__fr,Fy__fr,AM__fr] = pacejka_model(kappa__fr,Fz__fr,alpha__fr,gamma__fr,pacejkaParam);
[Fx__fl,Fy__fl,AM__fl] = pacejka_model(kappa__fl,Fz__fl,-alpha__fl,-gamma__fl,pacejkaParam);
% Now perform a second change of sign in order to restore the correct operating conditions
Fy__rl = -Fy__rl; AM__rl = -AM__rl;
Fy__fl = -Fy__fl; AM__fl = -AM__fl;
Mz_tires.rr = AM__rr;  Mz_tires.rl = AM__rl;  Mz_tires.fr = AM__fr;  Mz_tires.fl = AM__fl;

% ----------------------
% VERTICAL TIRE FORCES MODEL
% ----------------------
% Compute vertical tire loads
u_dot = dX_prev(4);
VerticalForces = LoadTransferModel(Omega,u,u_dot,FAz__r,FAz__f,Mz_tires,vehicle_data);
Fz__rr__ss = VerticalForces.Fz_rr_ss;
Fz__rl__ss = VerticalForces.Fz_rl_ss;
Fz__fr__ss = VerticalForces.Fz_fr_ss;
Fz__fl__ss = VerticalForces.Fz_fl_ss;

% ----------------------
% AXLE FORCES
% ----------------------
Fx__r = 0;  % ...
Fx__f = 0;  % ...
Fy__r = 0;  % ...
Fy__f = 0;  % ...
Delta__Fx__r = 0;  % ...
Delta__Fx__f = 0;  % ...

% ----------------------
% STEADY STATE SLIPS
% ----------------------
[kappa__rr__ss,kappa__rl__ss,kappa__fr__ss,kappa__fl__ss] = steadyStateLongSlips(omega__rr,omega__rl,omega__fr,omega__fl,Omega,u,delta__fr,delta__fl,vehicle_data);
[alpha__rr__ss,alpha__rl__ss,alpha__fr__ss,alpha__fl__ss] = steadyStateLatSlips(Omega,u,v,delta__fr,delta__fl,vehicle_data);


% ----------------------------------------------------------------
%% VEHICLE DATA
% ----------------------------------------------------------------
m      = vehicle_data.vehicle.m;
Lf     = vehicle_data.vehicle.Lf;
Lr     = vehicle_data.vehicle.Lr;
Wf     = vehicle_data.vehicle.Wf;
Wr     = vehicle_data.vehicle.Wr;
izz    = vehicle_data.vehicle.i_zz;
tau__N = vehicle_data.suspension.tau_N;
tau__D = vehicle_data.steering_system.tau_D;
tau__H = vehicle_data.steering_system.tau_H;
ly     = vehicle_data.vehicle.ly;
lx     = vehicle_data.vehicle.lx;
iwa__r = vehicle_data.rear_wheel.iwa_r;
iwa__f = vehicle_data.front_wheel.iwa_f;
Rr     = vehicle_data.rear_wheel.Rr;
Rf     = vehicle_data.front_wheel.Rf;
tau_ped = vehicle_data.motor.tau_ped;

% ----------------------------------------------------------------
%% VEHICLE MODEL DIFFERENTIAL EQUATIONS
% ----------------------------------------------------------------

% The following system of ODE is imported from Maple symbolic model

% Evolution of vehicle pose
x_dot        = u*cos(psi) - v*sin(psi);
y_dot        = v*cos(psi) + u*sin(psi);
psi_dot      = Omega;
% Newton equations
u_Dot        = 0;  % ...
v_Dot        = 0;  % ...
% Euler equation
Omega_Dot    = 0;  % ...
% Vertical loads first order dynamics
Fz_rr_Dot    = 0;  % ...
Fz_rl_Dot    = 0;  % ...
Fz_fr_Dot    = 0;  % ...
Fz_fl_Dot    = 0;  % ...
% Steering wheel first order dynamics
delta_Dot    = (-delta * tau__D + delta_req) / tau__D / tau__H;
% Side slip angle first order dynamics
alpha_rr_Dot = 0;  % ...
alpha_rl_Dot = 0;  % ...
alpha_fr_Dot = 0;  % ...
alpha_fl_Dot = 0;  % ...
% Longitudinal slip first order dynamics
kappa_rr_Dot = 0;  % ...
kappa_rl_Dot = 0;  % ...
kappa_fr_Dot = 0;  % ...
kappa_fl_Dot = 0;  % ...
% Wheel spin dynamics
omega_rr_Dot = 0;  % ...
omega_rl_Dot = 0;  % ...
omega_fr_Dot = 0;  % ...
omega_fl_Dot = 0;  % ...
% pedal dynamics
ped_Dot      = (pedal_req - ped) / tau_ped;

% Collect states derivatives in the dX vector
dX(1)  = x_dot;
dX(2)  = y_dot;
dX(3)  = psi_dot;
dX(4)  = u_Dot;
dX(5)  = v_Dot;
dX(6)  = Omega_Dot;
dX(7)  = Fz_rr_Dot;
dX(8)  = Fz_rl_Dot;
dX(9)  = Fz_fr_Dot;
dX(10) = Fz_fl_Dot;
dX(11) = delta_Dot;
dX(12) = omega_rr_Dot;
dX(13) = omega_rl_Dot;
dX(14) = omega_fr_Dot;
dX(15) = omega_fl_Dot;
dX(16) = alpha_rr_Dot;
dX(17) = alpha_rl_Dot;
dX(18) = alpha_fr_Dot;
dX(19) = alpha_fl_Dot;
dX(20) = kappa_rr_Dot;
dX(21) = kappa_rl_Dot;
dX(22) = kappa_fr_Dot;
dX(23) = kappa_fl_Dot;
dX(24) = ped_Dot;


% ----------------------------------------------------------------
%% SAVE USEFUL EXTRA PARAMETERS
% ----------------------------------------------------------------

extra_params(1)  = Tw__rr;
extra_params(2)  = Tw__rl;
extra_params(3)  = Tw__fr;
extra_params(4)  = Tw__fl;
extra_params(5)  = Fx__rr;
extra_params(6)  = Fx__rl;
extra_params(7)  = Fx__fr;
extra_params(8)  = Fx__fl;
extra_params(9)  = Fy__rr;
extra_params(10) = Fy__rl;
extra_params(11) = Fy__fr;
extra_params(12) = Fy__fl;
extra_params(13) = AM__rr;
extra_params(14) = AM__rl;
extra_params(15) = AM__fr;
extra_params(16) = AM__fl;
extra_params(17) = gamma__rr;
extra_params(18) = gamma__rl;
extra_params(19) = gamma__fr;
extra_params(20) = gamma__fl;
extra_params(21) = delta__fr;
extra_params(22) = delta__fl;

end

== matlab function framework_sim_r2018b/Lateral Controller/Arc Path Following Controller/Arc Path Following Controller ==
  data: target_Point input; delta output; pose input; endOfCircuit input
function delta  = arcPathFollowController(target_Point,pose,endOfCircuit)

    % Load vehicle params
    vehicle_params = getVehicleDataStruct();
    Lf = vehicle_params.vehicle.Lf;        
    Lr = vehicle_params.vehicle.Lr;    
    L  = Lf + Lr;  % [m] vehicle wheelbase
    
    % Current vehicle center of mass pose 
    x_C     = pose(1);
    y_C     = pose(2);
    theta_C = pose(3);  % vehicle attitude (in radians)
    
    %% COMPLETE THIS WITH YOUR CODE
    if (~endOfCircuit)
        delta = 0;    
    else
        delta = 0;
    end

end
